simulink library "DareLib"  (R2018b)
settings: Solver=VariableStepAuto  StartTime=0.0  StopTime=10.0  RelTol=1e-3
libraries: simulink x4, $bdroot x3
(part 1 of 2)
settings Model: Creator=zhaogl  LastModifiedBy=Administrator

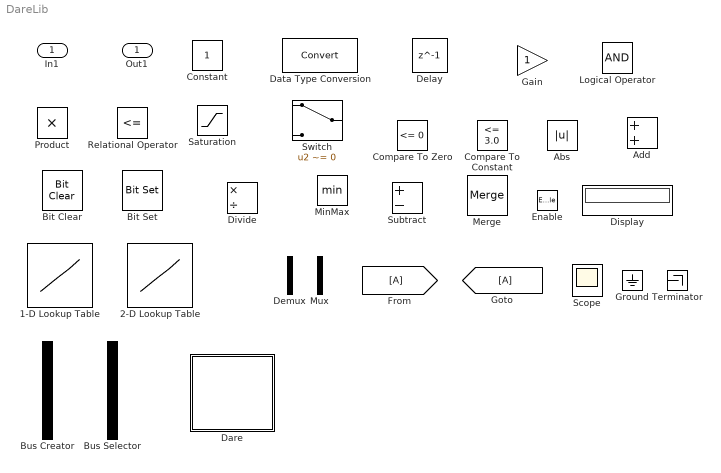
== system DareLib ==
  In1 : Inport
  Enable : EnablePort
      settings: AttributesFormatString=%<StatesWhenEnabling>
  1-D Lookup Table : Lookup_n-D  NumberOfTableDimensions=1  BreakpointsForDimension1=[-5:5]  Table=tanh([-5:5])  InternalRulePriority=Speed  RndMeth=Simplest  InputSameDT=on
  2-D Lookup Table : Lookup_n-D  BreakpointsForDimension1=[1:3]  BreakpointsForDimension2=[1:3]  InternalRulePriority=Speed  RndMeth=Simplest  InputSameDT=on
  Abs : Abs
  Add : Sum
  Bit Clear : simulink/Logic and Bit Operations/Bit Clear  iBit=0
      settings: SourceProductName=Simulink  SourceProductBaseCode=SL
  Bit Set : simulink/Logic and Bit Operations/Bit Set  iBit=0
      settings: SourceProductName=Simulink  SourceProductBaseCode=SL
  Bus Creator : BusCreator  Inputs=2
  Bus Selector : BusSelector  OutputSignals=signal1,signal2
  Compare To Constant : simulink/Logic and Bit Operations/Compare To Constant  relop=<=  const=3.0  OutDataTypeStr=boolean
  Compare To Zero : simulink/Logic and Bit Operations/Compare To Zero  relop=<=  OutDataTypeStr=boolean
  Constant : Constant
  Dare : Subsystem
      mask Display: image('Dare.jpg');
  Data Type Conversion : DataTypeConversion
  Delay : Delay  DelayLength=1  InitialCondition=0
  Demux : Demux  Outputs=2
  Display : Display
  Divide : Product  Inputs=*/
  Gain : Gain
  Ground : Ground
  Logical Operator : Logic  AllPortsSameDT=off  OutDataTypeStr=boolean
  Merge : Merge
  MinMax : MinMax
  Mux : Mux  Inputs=2
  Product : Product
  Relational Operator : RelationalOperator  Operator=<=  OutDataTypeStr=boolean  RndMeth=Simplest
  Saturation : Saturate
  Scope : Scope
  Subtract : Sum  Inputs=+-
  Switch : Switch  Criteria=u2 ~= 0
  Terminator : Terminator
  Out1 : Outport

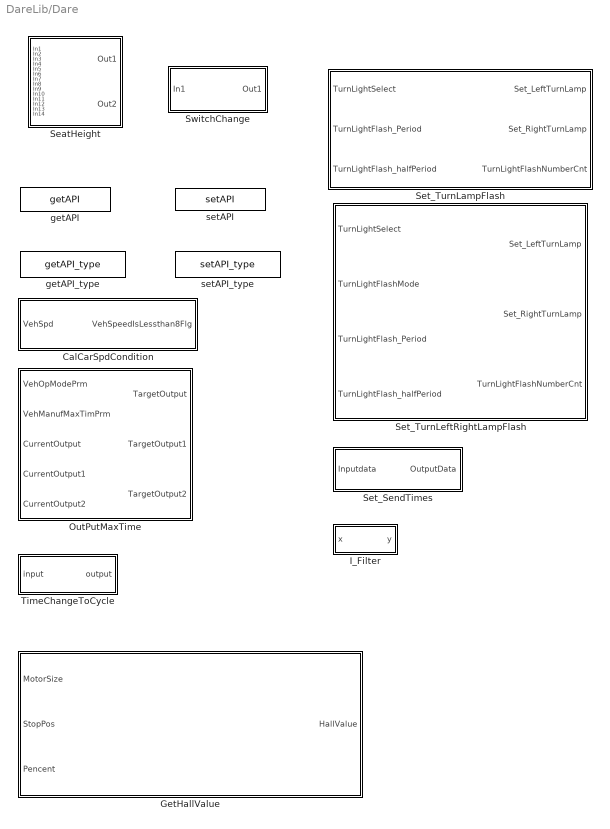
== system DareLib/Dare ==
  CalCarSpdCondition : Subsystem  mask(回差设定及判断){UpDeviationVal=9, DownDeviationVal=7, MaxOnTimer=500}
      mask prompts: UpDeviationVal "车速洄滞区间上限："; DownDeviationVal "车速洄滞区间下限："; MaxOnTimer "持续时间："
      mask help:
      | 功能描述
      | 车速判断回差，如雨刮速度模式的判断，当车速小于7km/h，持续时间5秒钟后，进入速度模式，大于9km/h持续时间5秒钟后退出速度模式，7~9km/h维持上次模式
      | 车速洄滞区间上限：如上述的9km/h
      | 车速洄滞区间下限：如上述的7km/h
      | 持续时间：如上述的5秒钟，需转成10ms单位，如5秒钟=5*1000/10=500
      mask Display:
      | port_label('input',1,'VehSpd','texmode','off');
      | 
      | 
      | port_label('output',1,'VehSpeedIsLessthan8Flg','texmode','off');
      | 
      | 
      | color('gray');
      | %disp('Dare');
      | text(0.14,0.8,'Dare','horizontalAlignment','right','verticalAlignment','bottom')
  GetHallValue : Subsystem
      settings: UndoDeleteFcn=Stateflow.SLINSF.SimulinkMan.restorePreDeleteFcn  PreDeleteFcn=Stateflow.SLINSF.SimulinkMan.removePreDeleteFcn
  I_Filter : Subsystem  mask(一阶滤波器){f=50}
      mask prompts: f "滤波系数："
      mask help: 用于信号滤波，滤波系数范围（0，100]，滤波系数越大，越接近输入值，滤波系数越小，曲线越平滑，根据实际需要选择不同滤波系数
      mask Display:
      | color('red');
      | disp(get_param(gcbh,'f'));
  OutPutMaxTime : Subsystem  Description=工厂模式限制输出时间  mask(OutPutMaxTime){UserMode=0, UnVaildValue=0}
      mask prompts: UserMode "用户模式值设定："; UnVaildValue "输出无效值设定："
      mask help: 在工厂模式和运输模式的最大工作时间设定，达到最大时间后输出无效值
      settings: AttributesFormatString=%<Description>
      mask Display:
      | port_label('input',1,'VehOpModePrm','texmode','off');
      | port_label('input',2,'VehManufMaxTimPrm','texmode','off');
      | port_label('input',3,'Input','texmode','off');
      | port_label('input',4,'Input1','texmode','off');
      | port_label('input',5,'Input2','texmode','off');
      | 
      | port_label('output',1,'Output','texmode','off');
      | port_label('output',2,'Output1','texmode','off');
      | port_label('output',3,'Output2','texmode','off');
      | 
      | 
      | color('gray')
      | text(0.11,0.94,'Dare','horizontalAlignment','right','verticalAlignment','bottom')
  SeatHeight : Subsystem
      mask help: 电动座椅控制封装函数
      mask Display: image('a.jpg');
  Set_SendTimes : Subsystem  mask(发送信号周期设定){Times=0}
      mask help:
      | InputSignal：输入发送信号
      | OnputSignal：输出发送信号
      | Times：设定发送信号不等于0时需要发送的帧数 (这实际是延迟周期数)，周期到后发送信号清零
      mask Display:
      | port_label('input',1,'InputSignal');
      | port_label('output',1,'OutputSignal');
      | 
      | color('gray');
      | %disp('Dare');
      | text(0.19,0.75,'Dare','horizontalAlignment','right','verticalAlignment','bottom')
  Set_TurnLampFlash : Subsystem  mask(控制转向灯闪烁及频率设定){TurnLight_Left=1, TurnLight_Right=2, TurnLight_LeftRight=3}
      mask prompts: TurnLight_Left "TurnLight_Left："; TurnLight_Right "TurnLight_Right："; TurnLight_LeftRight "TurnLight_LeftRight："
      mask help:
      | 第一个输入：TurnLightSelect：选择左右转向灯，enTurnLight_Left，enTurnLight_Right，enTurnLight_LeftRight
      | 第二个输入：TurnLightFlash_Period：闪烁周期设定
      | 第三个输入：TurnLightFlash_Period：闪烁周期内ON的时间设定
      | 参数设定，可根据实际修改：
      | TurnLight_Left：默认为1
      | TurnLight_Right：默认为2
      | TurnLight_LeftRight：默认为3
      mask Display:
      | port_label('input',1,'TurnLightSelect','texmode','off');
      | port_label('input',2,'TurnLightFlash_Period','texmode','off');
      | port_label('input',3,'TurnLightFlash_halfPeriod','texmode','off');
      | 
      | port_label('output',1,'Set_LeftTurnLamp','texmode','off');
      | port_label('output',2,'Set_RightTurnLamp','texmode','off');
      | port_label('output',3,'TurnLightFlashNumberCnt','texmode','off');
      | 
      | color('gray');
      | %disp('Dare');
      | text(0.09,0.93,'Dare','horizontalAlignment','right','verticalAlignment','bottom')
  Set_TurnLeftRightLampFlash : Subsystem  mask(控制转向灯闪烁频率设定及关闭){enTurnLight_Non=0, enTurnLight_Left=1, enTurnLight_Right=2, enTurnLight_LeftRight=3}
      mask prompts: enTurnLight_Non "TurnLight_Non"; enTurnLight_Left "TurnLight_Left"; enTurnLight_Right "TurnLight_Right"; enTurnLight_LeftRight "TurnLight_LeftRight"
      mask help:
      | 第一个输入：TurnLightSelect：选择左右转向灯，enTurnLight_Left，enTurnLight_Right，enTurnLight_LeftRight
      | 第二个输入：TurnLightFlashMode：ON为开启闪烁，OFF为关闭
      | 第三个输入：TurnLightFlash_Period：闪烁周期设定
      | 第四个输入：TurnLightFlash_Period：闪烁周期内ON的时间设定
      |
      | 参数设定：
      | enTurnLight_Non: 默认为0
      | enTurnLight_Left：默认为1
      | enTurnLight_Right：默认为2
      | enTurnLight_LeftRight：默认为3
      mask Display:
      | port_label('input',1,'TurnLightSelect','texmode','off');
      | port_label('input',2,'TurnLightFlashMode','texmode','off');
      | port_label('input',3,'TurnLightFlash_Period','texmode','off');
      | port_label('input',4,'TurnLightFlash_halfPeriod','texmode','off');
      | 
      | port_label('output',1,'Set_LeftTurnLamp','texmode','off');
      | port_label('output',2,'Set_RightTurnLamp','texmode','off');
      | port_label('output',3,'TurnLightFlashNumberCnt','texmode','off');
      | 
      | color('gray');
      | %disp('Dare');
      | text(0.12,0.96,'Dare','horizontalAlignment','right','verticalAlignment','bottom')
  SwitchChange : Subsystem  mask{d=1, a=0, b=1, c=2}
      mask prompts: d "设置开关有效："; a "状态  保持："; b "无效变有效："; c "有效变无效："
      mask help:
      | 检测自复位开关有效变化
      | 设置开关有效：如1有效则填1，2有效则填2
      mask Display:
      | disp('Reset Switch')
      | 
      | color('gray')
      | text(0.25,0.8,'Dare','horizontalAlignment','right','verticalAlignment','bottom')
  TimeChangeToCycle : Subsystem  Description=时间转成执行周期  mask{Sec=1, Msec=1000, Cycle=10}
      mask prompts: Sec "秒参数设定："; Msec "毫秒参数设定："; Cycle "执行周期设定："
      mask help:
      | y=x*sec*msec/cycle，通过时间计算执行周期
      | 秒参数设定：如果目标是分，填60s，如果目标是秒，填1，就是把分换算成秒
      | 毫秒参数设定：把秒换算成分，1s=1000ms
      | 执行周期设定：当前模型执行的周期
      settings: AttributesFormatString=%<Description>
      mask Display:
      | port_label('input',1,'input','texmode','off');
      | port_label('output',1,'output','texmode','off');
      | 
      | color('gray')
      | %disp('Dare');
      | text(0.25,0.75,'Dare','horizontalAlignment','right','verticalAlignment','bottom')
  getAPI : S-Function  FunctionName=getAPI  Parameters=g_funcname,g_param,g_type  SFunctionDeploymentMode=off  EnableBusSupport=off  mask(Dare Custom){g_funcname=getAPI, g_param=, g_type=uint8}
      mask prompts: g_funcname "API function name:"; g_param "API        param:"; g_type "API OutPut Type:"
      mask help:
      | This block generates get interface function API.
      | function name : Enter the interface function name.
      | param : Input interface function parameters
      | type :  choose The interface function returns the type
      settings: AttributesFormatString=%<g_funcname>
      mask TypeOptions g_type: boolean | uint8 | int8 | uint16 | int16 | uint32 | int32
      mask Display:
      | %color('green')
      | 
      | if isempty(g_param)
      |     %disp(get_param(gcbh,'g_funcname'));
      | else
      |     disp(get_param(gcbh,'g_param'));
      | end
      | %text(0.01,0.8,get_param(gcbh,'g_funcname'))
      | %text(0.6,0.2,get_param(gcbh,'g_param'))
      | 
      | color('gray')
      | text(0.25,0.63,'Dare','horizontalAlignment','right','verticalAlignment','bottom')
  getAPI_type : S-Function  FunctionName=getAPI_type  Parameters=g_funcname,g_param,g_type,g_enum,g_size  SFunctionDeploymentMode=off  EnableBusSupport=off  mask(Dare Custom){g_funcname=getAPI_type, g_param=, g_type=uint8, g_enum=, g_size=-1}
      mask prompts: g_funcname "API  Function Name:"; g_param "API  Param:"; g_type "API Output Type:"; g_enum "API Output Type Enum:"; g_size "API  Dimensions:"
      mask help:
      | This block generates get interface function API.
      | function name : Enter the interface function name.
      | param : Input interface function parameters
      | type :  choose The interface function returns the type
      | enum: choose enum type
      settings: AttributesFormatString=%<g_funcname>
      mask TypeOptions g_type: boolean | int8 | uint8 | int16 | uint16 | int32 | uint32 | double
      mask TypeOptions g_enum: ExitGearCause | enAdjustEnable | enBackGear | enDrAdjustEnable | enEngineType | enFinalPowerMode | enFrontGear | enHeatCmdFault | enHeatIoCmdLvl | enHeatIoSts | enHeatLvlSts | enHeatNtcFault | enHeatStopReason | enHeatType | enIgnSts | enLearnCmd | enLearnExitCause | enLearnSts | enLengthGear | enMasReason | enMassageLevel_DSM | enMassageLevel_IVI | enMassageMode_DSM | enMassageMode_IVI | enMemBtn | enMemCallFb | enMemSet | enMemSetFb | enMemStopCause | enMotorLearn | enNapMode | enPowerModeSts | enProjectType | enResCallRet | enResetSts | enSWMoveCmd | enSeatAutoRunSts | enSeatHightMotorRunsts | enSeatMemBtnCmd | enSeatMemBtnSts | enSeatMemStsAndMsg | enSeatMemStsFb | enSeatMotorRunTye | enSeatMotorRunType | enSeatMoveCmd | enSoftStopFault | enSteerHeatType | enSystemVolt | enTcmGearLvlSts | enVehTypePrm | enVehicleRunType | enVentCmdFault | enVentIoCmdLvl | enVentLvlSts | enVentStopReason | enVentType | enVoltageMode | enWelStopCause | enWelcomeRunSts | enWelcomeSts
      mask Display:
      | %color('green')
      | 
      | if isempty(g_param)
      |     %disp(get_param(gcbh,'g_funcname'));
      | else
      |     disp(get_param(gcbh,'g_param'));
      | end
      | %text(0.01,0.8,get_param(gcbh,'g_funcname'))
      | %text(0.6,0.2,get_param(gcbh,'g_param'))
      | 
      | color('gray')
      | text(0.25,0.63,'Dare','horizontalAlignment','right','verticalAlignment','bottom')
      | 
      | if isempty(get_param(gcbh,'g_enum'))
      |     set_param(gcbh','MaskVisibilityString', 'on,on,on,on,on')
      | else
      |     set_param(gcbh','MaskVisibilityString', 'on,on,off,on,on')
      | end
  setAPI : S-Function  FunctionName=setAPI  Parameters=g_funcname,g_param,g_type  SFunctionDeploymentMode=off  EnableBusSupport=off  mask(Dare Custom){g_funcname=setAPI, g_param=, g_type=uint8}
      mask prompts: g_funcname "API function name:"; g_param "API         param:"; g_type "API OutPut Type:"
      mask help:
      | This block generates set interface function API.
      | function name : Enter the interface function name.
      | API function param : Input interface function parameters
      | API param：choose channel number
      | type :  choose The interface function returns the type
      settings: AttributesFormatString=%<g_funcname>
      mask TypeOptions g_type: boolean | uint8 | int8 | uint16 | int16 | uint32 | int32 | double
      mask Display:
      | %color('magenta')
      | %disp(get_param(gcbh,'g_param'))
      | if isempty(g_param)
      |     %disp(get_param(gcbh,'g_funcname'));
      | else
      |     disp(get_param(gcbh,'g_param'));
      | end
      | 
      | color('gray')
      | text(0.25,0.61,'Dare','horizontalAlignment','right','verticalAlignment','bottom')
  setAPI_type : S-Function  FunctionName=setAPI_type  Parameters=g_funcname,g_param,g_type,g_enum,g_size  SFunctionDeploymentMode=off  EnableBusSupport=off  mask(Dare Custom){g_funcname=setAPI_type, g_param=, g_type=uint8, g_enum=, g_size=-1}
      mask prompts: g_funcname "API  Function Name:"; g_param "API  Param:"; g_type "API Output Type:"; g_enum "API Output Type Enum:"; g_size "API  Dimensions:"
      mask help:
      | This block generates get interface function API.
      | function name : Enter the interface function name.
      | param : Input interface function parameters
      | type :  choose The interface function returns the type
      | enum: choose enum type
      settings: AttributesFormatString=%<g_funcname>
      mask TypeOptions g_type: boolean | int8 | uint8 | int16 | uint16 | int32 | uint32 | double
      mask TypeOptions g_enum: ExitGearCause | enAdjustEnable | enBackGear | enDrAdjustEnable | enEngineType | enFinalPowerMode | enFrontGear | enHeatCmdFault | enHeatIoCmdLvl | enHeatIoSts | enHeatLvlSts | enHeatNtcFault | enHeatStopReason | enHeatType | enIgnSts | enLearnCmd | enLearnExitCause | enLearnSts | enLengthGear | enMasReason | enMassageLevel_DSM | enMassageLevel_IVI | enMassageMode_DSM | enMassageMode_IVI | enMemBtn | enMemCallFb | enMemSet | enMemSetFb | enMemStopCause | enMotorLearn | enNapMode | enPowerModeSts | enProjectType | enResCallRet | enResetSts | enSWMoveCmd | enSeatAutoRunSts | enSeatHightMotorRunsts | enSeatMemBtnCmd | enSeatMemBtnSts | enSeatMemStsAndMsg | enSeatMemStsFb | enSeatMotorRunTye | enSeatMotorRunType | enSeatMoveCmd | enSoftStopFault | enSteerHeatType | enSystemVolt | enTcmGearLvlSts | enVehTypePrm | enVehicleRunType | enVentCmdFault | enVentIoCmdLvl | enVentLvlSts | enVentStopReason | enVentType | enVoltageMode | enWelStopCause | enWelcomeRunSts | enWelcomeSts
      mask Display:
      | %color('green')
      | 
      | if isempty(get_param(gcbh,'g_param'))
      |     %disp(get_param(gcbh,'g_funcname'));
      | else
      |     disp(get_param(gcbh,'g_param'));
      | end
      | %text(0.01,0.8,get_param(gcbh,'g_funcname'))
      | %text(0.6,0.2,get_param(gcbh,'g_param'))
      | 
      | color('gray')
      | text(0.25,0.63,'Dare','horizontalAlignment','right','verticalAlignment','bottom')
      | 
      | if isempty(get_param(gcbh,'g_enum'))
      |     set_param(gcbh','MaskVisibilityString', 'on,on,on,on,on')
      | else
      |     set_param(gcbh','MaskVisibilityString', 'on,on,off,on,on')
      | end

== system DareLib/Dare/CalCarSpdCondition ==
  " VehSpd" : Inport
  Chart : Stateflow chart  TreatAsAtomicUnit=on
  Constant : Constant  Value=UpDeviationVal  OutDataTypeStr=uint8
  Constant2 : Constant  Value=DownDeviationVal  OutDataTypeStr=uint8
  Constant3 : Constant  Value=MaxOnTimer  OutDataTypeStr=uint16
  VehSpeedIsLessthan8Flg : Outport
  wires:
  " VehSpd"/1 -> Chart/1(VehSpd)
  Constant3/1 -> Chart/4(CAL_MaxOnTimer)
  Chart/1(VehSpdUpDnFlg) -> VehSpeedIsLessthan8Flg/1
  Constant/1 -> Chart/3(UpVal)
  Constant2/1 -> Chart/2(DnVal)

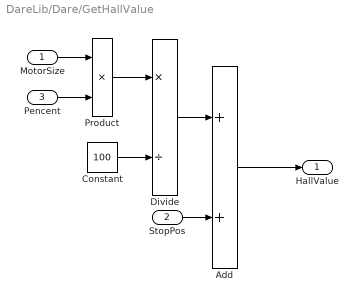
== system DareLib/Dare/GetHallValue ==
  MotorSize : Inport  OutDataTypeStr=uint16
  StopPos : Inport  Port=2  OutDataTypeStr=uint16
  Pencent : Inport  Port=3  OutDataTypeStr=uint8
  Add : Sum  AccumDataTypeStr=uint16
  Constant : Constant  Value=100  OutDataTypeStr=uint16
  Divide : Product  Inputs=*/  OutDataTypeStr=uint16
  Product : Product  OutDataTypeStr=uint32
  HallValue : Outport  OutDataTypeStr=uint16
  wires:
  Divide/1 -> Add/1
  Constant/1 -> Divide/2
  Product/1 -> Divide/1
  Pencent/1 -> Product/2
  StopPos/1 -> Add/2
  MotorSize/1 -> Product/1
  Add/1 -> HallValue/1

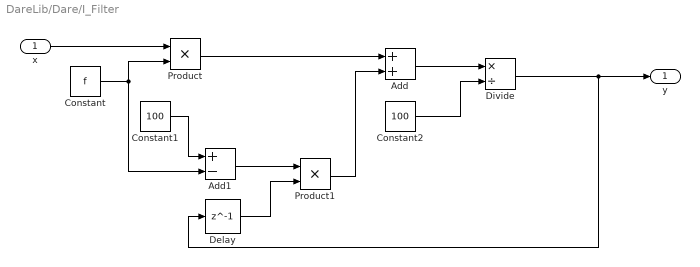
== system DareLib/Dare/I_Filter ==
  x : Inport
  Add : Sum
  Add1 : Sum  Inputs=+-
  Constant : Constant  Value=f  OutDataTypeStr=uint8
  Constant1 : Constant  Value=100  OutDataTypeStr=uint8
  Constant2 : Constant  Value=100  OutDataTypeStr=uint8
  Delay : Delay  DelayLength=1  InitialCondition=0
  Divide : Product  Inputs=*/
  Product : Product
  Product1 : Product  OutDataTypeStr=uint32
  y : Outport
  wires:
  Constant2/1 -> Divide/2
  Add/1 -> Divide/1
  Add1/1 -> Product1/1
  Product/1 -> Add/1
  Delay/1 -> Product1/2
  Product1/1 -> Add/2
  Divide/1 -> Delay/1, y/1
  x/1 -> Product/1
  Constant1/1 -> Add1/1
  Constant/1 -> Product/2, Add1/2

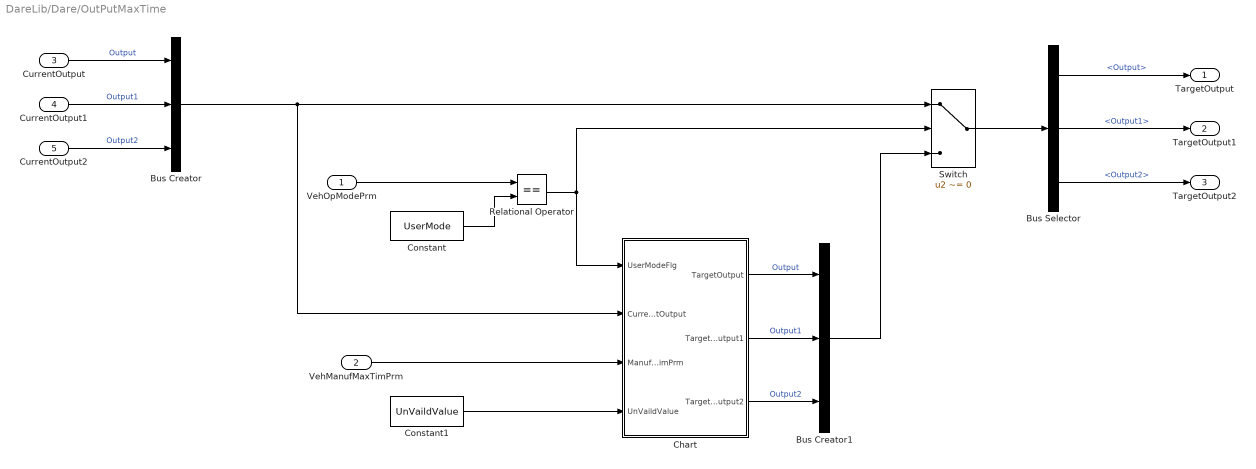
== system DareLib/Dare/OutPutMaxTime ==
  VehOpModePrm : Inport
  VehManufMaxTimPrm : Inport  Port=2
  CurrentOutput : Inport  Port=3
  CurrentOutput1 : Inport  Port=4
  CurrentOutput2 : Inport  Port=5
  Bus Creator : BusCreator  Inputs=3
  Bus Creator1 : BusCreator  Inputs=3
  Bus Selector : BusSelector  OutputSignals=Output,Output1,Output2
  Chart : Stateflow chart  TreatAsAtomicUnit=on
  Constant : Constant  Value=UserMode  OutDataTypeStr=uint8
  Constant1 : Constant  Value=UnVaildValue  OutDataTypeStr=uint8
  Relational Operator : RelationalOperator  Operator===  OutDataTypeStr=boolean  RndMeth=Simplest
  Switch : Switch  Criteria=u2 ~= 0
  TargetOutput : Outport
  TargetOutput1 : Outport  Port=2
  TargetOutput2 : Outport  Port=3
  wires:
  Constant1/1 -> Chart/4(UnVaildValue)
  Relational Operator/1 -> Chart/1(UserModeFlg), Switch/2
  VehManufMaxTimPrm/1 -> Chart/3(ManufMaxTimPrm)
  Constant/1 -> Relational Operator/2
  Bus Creator/1 -> Chart/2(CurrentOutput), Switch/1
  VehOpModePrm/1 -> Relational Operator/1
  CurrentOutput/1 -> Bus Creator/1  "Output"
  CurrentOutput1/1 -> Bus Creator/2  "Output1"
  CurrentOutput2/1 -> Bus Creator/3  "Output2"
  Chart/3(TargetOutput2) -> Bus Creator1/3  "Output2"
  Chart/1(TargetOutput) -> Bus Creator1/1  "Output"
  Bus Creator1/1 -> Switch/3
  Chart/2(TargetOutput1) -> Bus Creator1/2  "Output1"
  Bus Selector/2 -> TargetOutput1/1  "<Output1>"
  Bus Selector/1 -> TargetOutput/1  "<Output>"
  Switch/1 -> Bus Selector/1
  Bus Selector/3 -> TargetOutput2/1  "<Output2>"

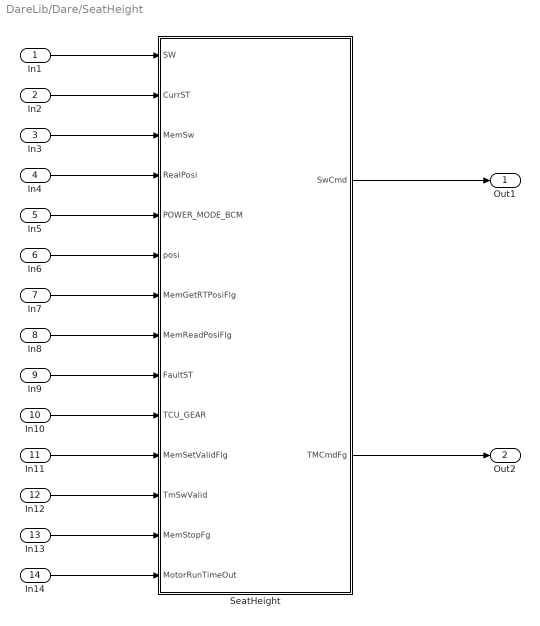
== system DareLib/Dare/SeatHeight ==
  In1 : Inport
  In2 : Inport  Port=2
  In3 : Inport  Port=3
  In4 : Inport  Port=4
  In5 : Inport  Port=5
  In6 : Inport  Port=6
  In7 : Inport  Port=7
  In8 : Inport  Port=8
  In9 : Inport  Port=9
  In10 : Inport  Port=10
  In11 : Inport  Port=11
  In12 : Inport  Port=12
  In13 : Inport  Port=13
  In14 : Inport  Port=14
  SeatHeight : Stateflow chart  TreatAsAtomicUnit=on
  Out1 : Outport
  Out2 : Outport  Port=2
  wires:
  In4/1 -> SeatHeight/4(RealPosi)
  In5/1 -> SeatHeight/5(POWER_MODE_BCM)
  In7/1 -> SeatHeight/7(MemGetRTPosiFlg)
  In8/1 -> SeatHeight/8(MemReadPosiFlg)
  SeatHeight/1(SwCmd) -> Out1/1
  In3/1 -> SeatHeight/3(MemSw)
  In6/1 -> SeatHeight/6(posi)
  In1/1 -> SeatHeight/1(SW)
  In9/1 -> SeatHeight/9(FaultST)
  In2/1 -> SeatHeight/2(CurrST)
  In12/1 -> SeatHeight/12(TmSwValid)
  In10/1 -> SeatHeight/10(TCU_GEAR)
  In11/1 -> SeatHeight/11(MemSetValidFlg)
  In14/1 -> SeatHeight/14(MotorRunTimeOut)
  In13/1 -> SeatHeight/13(MemStopFg)
  SeatHeight/2(TMCmdFg) -> Out2/1

== system DareLib/Dare/Set_SendTimes ==
  Inputdata : Inport
  Chart : Stateflow chart  TreatAsAtomicUnit=on
  Times : Constant  Value=Times  OutDataTypeStr=uint8
  OutputData : Outport
  wires:
  Inputdata/1 -> Chart/1(Inputdata)
  Times/1 -> Chart/2(Times)
  Chart/1(OutputData) -> OutputData/1

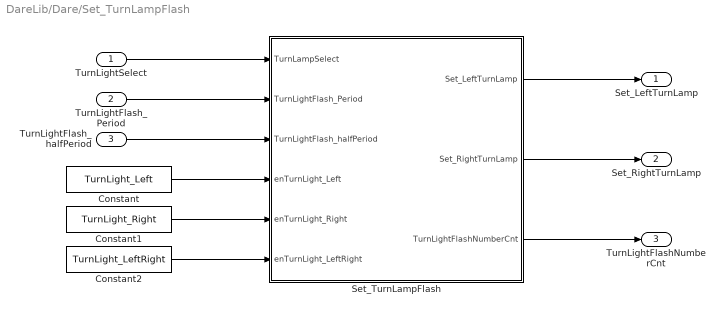
== system DareLib/Dare/Set_TurnLampFlash ==
  TurnLightSelect : Inport
  TurnLightFlash_Period : Inport  Port=2
  TurnLightFlash_halfPeriod : Inport  Port=3
  Constant : Constant  Value=TurnLight_Left  OutDataTypeStr=uint8
  Constant1 : Constant  Value=TurnLight_Right  OutDataTypeStr=uint8
  Constant2 : Constant  Value=TurnLight_LeftRight  OutDataTypeStr=uint8
  Set_TurnLampFlash : Stateflow chart  TreatAsAtomicUnit=on
  Set_LeftTurnLamp : Outport
  Set_RightTurnLamp : Outport  Port=2
  TurnLightFlashNumberCnt : Outport  Port=3
  wires:
  Constant/1 -> Set_TurnLampFlash/4(enTurnLight_Left)
  Constant1/1 -> Set_TurnLampFlash/5(enTurnLight_Right)
  Constant2/1 -> Set_TurnLampFlash/6(enTurnLight_LeftRight)
  TurnLightFlash_Period/1 -> Set_TurnLampFlash/2(TurnLightFlash_Period)
  Set_TurnLampFlash/2(Set_RightTurnLamp) -> Set_RightTurnLamp/1
  Set_TurnLampFlash/1(Set_LeftTurnLamp) -> Set_LeftTurnLamp/1
  TurnLightSelect/1 -> Set_TurnLampFlash/1(TurnLampSelect)
  TurnLightFlash_halfPeriod/1 -> Set_TurnLampFlash/3(TurnLightFlash_halfPeriod)
  Set_TurnLampFlash/3(TurnLightFlashNumberCnt) -> TurnLightFlashNumberCnt/1

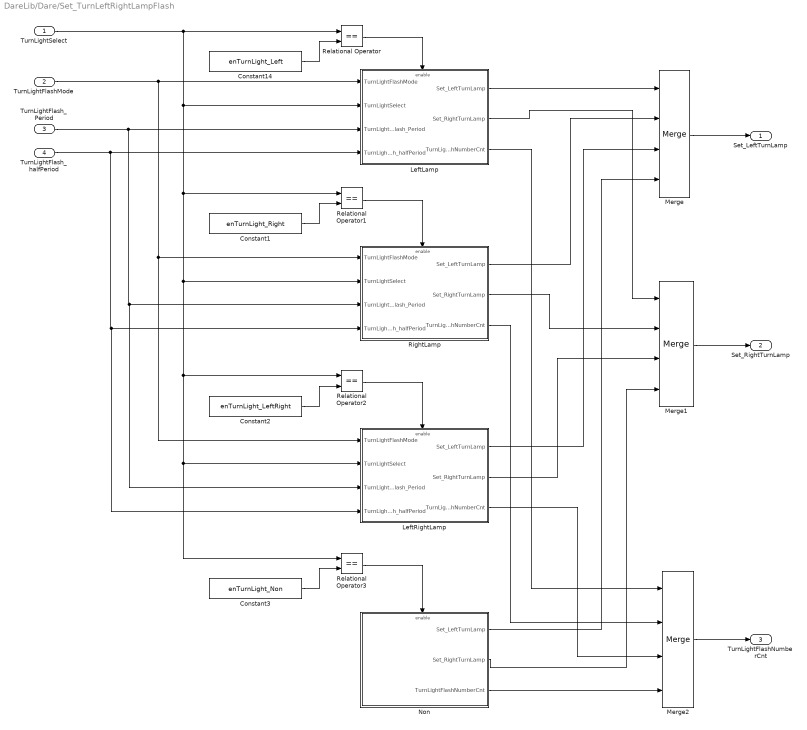
== system DareLib/Dare/Set_TurnLeftRightLampFlash ==
  TurnLightSelect : Inport
  TurnLightFlashMode : Inport  Port=2
  TurnLightFlash_Period : Inport  Port=3
  TurnLightFlash_halfPeriod : Inport  Port=4
  Constant1 : Constant  Value=enTurnLight_Right  OutDataTypeStr=uint8
  Constant14 : Constant  Value=enTurnLight_Left  OutDataTypeStr=uint8
  Constant2 : Constant  Value=enTurnLight_LeftRight  OutDataTypeStr=uint8
  Constant3 : Constant  Value=enTurnLight_Non  OutDataTypeStr=uint8
  LeftLamp : Subsystem  TreatAsAtomicUnit=on
  LeftRightLamp : Subsystem  TreatAsAtomicUnit=on
  Merge : Merge  Inputs=4
  Merge1 : Merge  Inputs=4
  Merge2 : Merge  Inputs=4
  Non : Subsystem  TreatAsAtomicUnit=on
  Relational Operator{,1..3} (4 alike) : RelationalOperator  Operator===  OutDataTypeStr=boolean  RndMeth=Simplest
  RightLamp : Subsystem  TreatAsAtomicUnit=on
  Set_LeftTurnLamp : Outport
  Set_RightTurnLamp : Outport  Port=2
  TurnLightFlashNumberCnt : Outport  Port=3
  wires:
  LeftLamp/2(Set_RightTurnLamp) -> Merge1/1
  Relational Operator1/1 -> RightLamp/Enable
  Constant1/1 -> Relational Operator1/2
  Relational Operator/1 -> LeftLamp/Enable
  RightLamp/3(TurnLightFlashNumberCnt) -> Merge2/2
  Constant14/1 -> Relational Operator/2
  Constant2/1 -> Relational Operator2/2
  Relational Operator2/1 -> LeftRightLamp/Enable
  LeftLamp/3(TurnLightFlashNumberCnt) -> Merge2/1
  RightLamp/2(Set_RightTurnLamp) -> Merge1/2
  LeftRightLamp/1(Set_LeftTurnLamp) -> Merge/3
  Merge/1 -> Set_LeftTurnLamp/1
  Merge1/1 -> Set_RightTurnLamp/1
  LeftLamp/1(Set_LeftTurnLamp) -> Merge/1
  LeftRightLamp/2(Set_RightTurnLamp) -> Merge1/3
  LeftRightLamp/3(TurnLightFlashNumberCnt) -> Merge2/3
  Merge2/1 -> TurnLightFlashNumberCnt/1
  RightLamp/1(Set_LeftTurnLamp) -> Merge/2
  TurnLightFlash_Period/1 -> LeftRightLamp/3(TurnLightFlash_Period), RightLamp/3(TurnLightFlash_Period), LeftLamp/3(TurnLightFlash_Period)
  Relational Operator3/1 -> Non/Enable
  Constant3/1 -> Relational Operator3/2
  TurnLightFlash_halfPeriod/1 -> LeftRightLamp/4(TurnLightFlash_halfPeriod), RightLamp/4(TurnLightFlash_halfPeriod), LeftLamp/4(TurnLightFlash_halfPeriod)
  TurnLightSelect/1 -> LeftLamp/2(TurnLightSelect), RightLamp/2(TurnLightSelect), Relational Operator3/1, LeftRightLamp/2(TurnLightSelect), Relational Operator2/1, Relational Operator1/1, Relational Operator/1
  TurnLightFlashMode/1 -> LeftRightLamp/1(TurnLightFlashMode), RightLamp/1(TurnLightFlashMode), LeftLamp/1(TurnLightFlashMode)
  Non/3(TurnLightFlashNumberCnt) -> Merge2/4
  Non/1(Set_LeftTurnLamp) -> Merge/4
  Non/2(Set_RightTurnLamp) -> Merge1/4

== system DareLib/Dare/SwitchChange ==
  In1 : Inport
  ButtonChange : Stateflow chart  TreatAsAtomicUnit=on
  Constant1 : Constant  Value=d  OutDataTypeStr=uint8
  Constant2 : Constant  Value=a  OutDataTypeStr=uint8
  Constant3 : Constant  Value=b  OutDataTypeStr=uint8
  Constant4 : Constant  Value=c  OutDataTypeStr=uint8
  Out1 : Outport
  wires:
  Constant2/1 -> ButtonChange/2(enSw_NoChanged)
  In1/1 -> ButtonChange/1(CurSw)
  Constant4/1 -> ButtonChange/4(enSw_ValidToUnvalid)
  Constant3/1 -> ButtonChange/3(enSw_UnvalidToValid)
  ButtonChange/1(SwSts) -> Out1/1
  Constant1/1 -> ButtonChange/5(Vaild_Vaule)

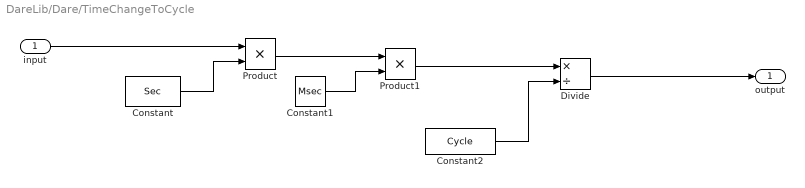
== system DareLib/Dare/TimeChangeToCycle ==
  input : Inport
  Constant : Constant  Value=Sec  OutDataTypeStr=uint16
  Constant1 : Constant  Value=Msec  OutDataTypeStr=uint16
  Constant2 : Constant  Value=Cycle  OutDataTypeStr=uint8
  Divide : Product  Inputs=*/  OutDataTypeStr=uint32
  Product : Product
  Product1 : Product  OutDataTypeStr=uint32
  output : Outport
  wires:
  Constant2/1 -> Divide/2
  Product/1 -> Product1/1
  Constant1/1 -> Product1/2
  Product1/1 -> Divide/1
  Constant/1 -> Product/2
  input/1 -> Product/1
  Divide/1 -> output/1

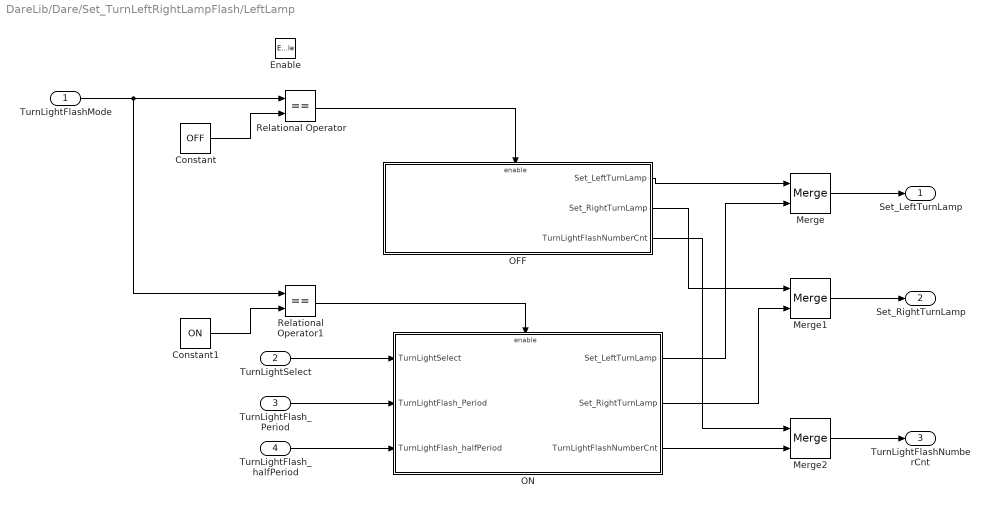
== system DareLib/Dare/Set_TurnLeftRightLampFlash/LeftLamp ==
  TurnLightFlashMode : Inport
  TurnLightSelect : Inport  Port=2
  TurnLightFlash_Period : Inport  Port=3
  TurnLightFlash_halfPeriod : Inport  Port=4
  Enable : EnablePort
  Constant : Constant  Value=OFF  OutDataTypeStr=uint8
  Constant1 : Constant  Value=ON  OutDataTypeStr=uint8
  Merge : Merge
  Merge1 : Merge
  Merge2 : Merge
  OFF : Subsystem  TreatAsAtomicUnit=on
  ON : Subsystem  TreatAsAtomicUnit=on
  Relational Operator : RelationalOperator  Operator===  OutDataTypeStr=boolean  RndMeth=Simplest
  Relational Operator1 : RelationalOperator  Operator===  OutDataTypeStr=boolean  RndMeth=Simplest
  Set_LeftTurnLamp : Outport
  Set_RightTurnLamp : Outport  Port=2
  TurnLightFlashNumberCnt : Outport  Port=3
  wires:
  Relational Operator/1 -> OFF/Enable
  Constant/1 -> Relational Operator/2
  Constant1/1 -> Relational Operator1/2
  Relational Operator1/1 -> ON/Enable
  TurnLightFlashMode/1 -> Relational Operator1/1, Relational Operator/1
  OFF/1(Set_LeftTurnLamp) -> Merge/1
  ON/1(Set_LeftTurnLamp) -> Merge/2
  OFF/2(Set_RightTurnLamp) -> Merge1/1
  ON/2(Set_RightTurnLamp) -> Merge1/2
  Merge/1 -> Set_LeftTurnLamp/1
  Merge1/1 -> Set_RightTurnLamp/1
  TurnLightSelect/1 -> ON/1(TurnLightSelect)
  TurnLightFlash_Period/1 -> ON/2(TurnLightFlash_Period)
  TurnLightFlash_halfPeriod/1 -> ON/3(TurnLightFlash_halfPeriod)
  Merge2/1 -> TurnLightFlashNumberCnt/1
  OFF/3(TurnLightFlashNumberCnt) -> Merge2/1
  ON/3(TurnLightFlashNumberCnt) -> Merge2/2

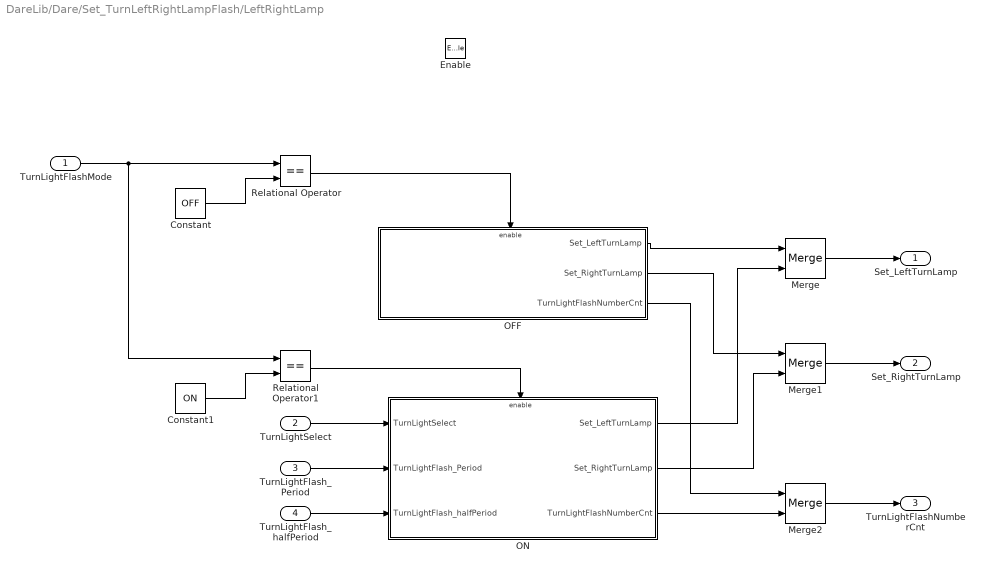
== system DareLib/Dare/Set_TurnLeftRightLampFlash/LeftRightLamp ==
  TurnLightFlashMode : Inport
  TurnLightSelect : Inport  Port=2
  TurnLightFlash_Period : Inport  Port=3
  TurnLightFlash_halfPeriod : Inport  Port=4
  Enable : EnablePort
  Constant : Constant  Value=OFF
  Constant1 : Constant  Value=ON
  Merge : Merge
  Merge1 : Merge
  Merge2 : Merge
  OFF : Subsystem  TreatAsAtomicUnit=on
  ON : Subsystem  TreatAsAtomicUnit=on
  Relational Operator : RelationalOperator  Operator===  OutDataTypeStr=boolean  RndMeth=Simplest
  Relational Operator1 : RelationalOperator  Operator===  OutDataTypeStr=boolean  RndMeth=Simplest
  Set_LeftTurnLamp : Outport
  Set_RightTurnLamp : Outport  Port=2
  TurnLightFlashNumberCnt : Outport  Port=3
  wires:
  Constant/1 -> Relational Operator/2
  Relational Operator1/1 -> ON/Enable
  Relational Operator/1 -> OFF/Enable
  Constant1/1 -> Relational Operator1/2
  TurnLightFlashMode/1 -> Relational Operator1/1, Relational Operator/1
  Merge/1 -> Set_LeftTurnLamp/1
  ON/2(Set_RightTurnLamp) -> Merge1/2
  OFF/1(Set_LeftTurnLamp) -> Merge/1
  OFF/2(Set_RightTurnLamp) -> Merge1/1
  Merge1/1 -> Set_RightTurnLamp/1
  ON/1(Set_LeftTurnLamp) -> Merge/2
  TurnLightSelect/1 -> ON/1(TurnLightSelect)
  TurnLightFlash_Period/1 -> ON/2(TurnLightFlash_Period)
  TurnLightFlash_halfPeriod/1 -> ON/3(TurnLightFlash_halfPeriod)
  ON/3(TurnLightFlashNumberCnt) -> Merge2/2
  OFF/3(TurnLightFlashNumberCnt) -> Merge2/1
  Merge2/1 -> TurnLightFlashNumberCnt/1

== system DareLib/Dare/Set_TurnLeftRightLampFlash/Non ==
  Enable : EnablePort
  Constant : Constant  Value=0  OutDataTypeStr=uint8
  Constant1 : Constant  Value=0  OutDataTypeStr=uint8
  Constant2 : Constant  Value=0  OutDataTypeStr=uint16
  Set_LeftTurnLamp : Outport
  Set_RightTurnLamp : Outport  Port=2
  TurnLightFlashNumberCnt : Outport  Port=3
  wires:
  Constant1/1 -> Set_RightTurnLamp/1
  Constant/1 -> Set_LeftTurnLamp/1
  Constant2/1 -> TurnLightFlashNumberCnt/1

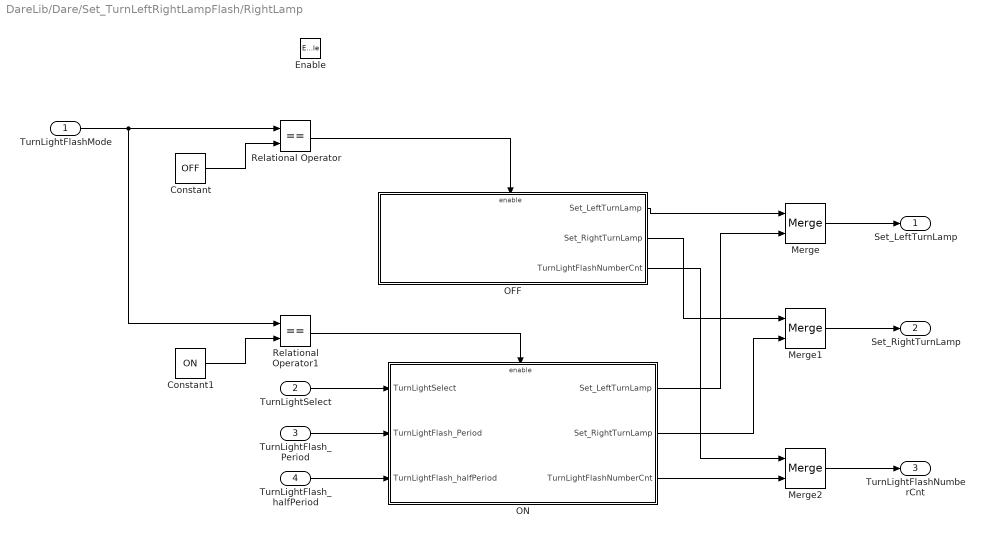
== system DareLib/Dare/Set_TurnLeftRightLampFlash/RightLamp ==
  TurnLightFlashMode : Inport
  TurnLightSelect : Inport  Port=2
  TurnLightFlash_Period : Inport  Port=3
  TurnLightFlash_halfPeriod : Inport  Port=4
  Enable : EnablePort
  Constant : Constant  Value=OFF
  Constant1 : Constant  Value=ON
  Merge : Merge
  Merge1 : Merge
  Merge2 : Merge
  OFF : Subsystem  TreatAsAtomicUnit=on
  ON : Subsystem  TreatAsAtomicUnit=on
  Relational Operator : RelationalOperator  Operator===  OutDataTypeStr=boolean  RndMeth=Simplest
  Relational Operator1 : RelationalOperator  Operator===  OutDataTypeStr=boolean  RndMeth=Simplest
  Set_LeftTurnLamp : Outport
  Set_RightTurnLamp : Outport  Port=2
  TurnLightFlashNumberCnt : Outport  Port=3
  wires:
  TurnLightFlashMode/1 -> Relational Operator1/1, Relational Operator/1
  Relational Operator1/1 -> ON/Enable
  Constant1/1 -> Relational Operator1/2
  Constant/1 -> Relational Operator/2
  Relational Operator/1 -> OFF/Enable
  Merge/1 -> Set_LeftTurnLamp/1
  ON/2(Set_RightTurnLamp) -> Merge1/2
  OFF/1(Set_LeftTurnLamp) -> Merge/1
  OFF/2(Set_RightTurnLamp) -> Merge1/1
  Merge1/1 -> Set_RightTurnLamp/1
  ON/1(Set_LeftTurnLamp) -> Merge/2
  TurnLightSelect/1 -> ON/1(TurnLightSelect)
  TurnLightFlash_Period/1 -> ON/2(TurnLightFlash_Period)
  TurnLightFlash_halfPeriod/1 -> ON/3(TurnLightFlash_halfPeriod)
  Merge2/1 -> TurnLightFlashNumberCnt/1
  OFF/3(TurnLightFlashNumberCnt) -> Merge2/1
  ON/3(TurnLightFlashNumberCnt) -> Merge2/2

== system DareLib/Dare/Set_TurnLeftRightLampFlash/LeftLamp/OFF ==
  Enable : EnablePort
  Constant : Constant  Value=0  OutDataTypeStr=uint8
  Constant1 : Constant  Value=0  OutDataTypeStr=uint8
  Constant2 : Constant  Value=0  OutDataTypeStr=uint16
  Set_LeftTurnLamp : Outport
  Set_RightTurnLamp : Outport  Port=2
  TurnLightFlashNumberCnt : Outport  Port=3
  wires:
  Constant/1 -> Set_LeftTurnLamp/1
  Constant1/1 -> Set_RightTurnLamp/1
  Constant2/1 -> TurnLightFlashNumberCnt/1

== system DareLib/Dare/Set_TurnLeftRightLampFlash/LeftLamp/ON ==
  TurnLightSelect : Inport
  TurnLightFlash_Period : Inport  Port=2
  TurnLightFlash_halfPeriod : Inport  Port=3
  Enable : EnablePort  StatesWhenEnabling=reset
      settings: AttributesFormatString=%<StatesWhenEnabling>
  Set_TurnLampFlash : $bdroot/Dare/Set_TurnLampFlash  TurnLight_Left=1  TurnLight_Right=2  TurnLight_LeftRight=3
  Set_LeftTurnLamp : Outport
  Set_RightTurnLamp : Outport  Port=2
  TurnLightFlashNumberCnt : Outport  Port=3
  wires:
  TurnLightSelect/1 -> Set_TurnLampFlash/1
  TurnLightFlash_Period/1 -> Set_TurnLampFlash/2
  TurnLightFlash_halfPeriod/1 -> Set_TurnLampFlash/3
  Set_TurnLampFlash/1 -> Set_LeftTurnLamp/1
  Set_TurnLampFlash/2 -> Set_RightTurnLamp/1
  Set_TurnLampFlash/3 -> TurnLightFlashNumberCnt/1

== system DareLib/Dare/Set_TurnLeftRightLampFlash/LeftRightLamp/OFF ==
  Enable : EnablePort
  Constant : Constant  Value=0  OutDataTypeStr=uint8
  Constant1 : Constant  Value=0  OutDataTypeStr=uint8
  Constant2 : Constant  Value=0  OutDataTypeStr=uint16
  Set_LeftTurnLamp : Outport
  Set_RightTurnLamp : Outport  Port=2
  TurnLightFlashNumberCnt : Outport  Port=3
  wires:
  Constant/1 -> Set_LeftTurnLamp/1
  Constant1/1 -> Set_RightTurnLamp/1
  Constant2/1 -> TurnLightFlashNumberCnt/1

== system DareLib/Dare/Set_TurnLeftRightLampFlash/LeftRightLamp/ON ==
  TurnLightSelect : Inport
  TurnLightFlash_Period : Inport  Port=2
  TurnLightFlash_halfPeriod : Inport  Port=3
  Enable : EnablePort  StatesWhenEnabling=reset
      settings: AttributesFormatString=%<StatesWhenEnabling>
  Set_TurnLampFlash : $bdroot/Dare/Set_TurnLampFlash  TurnLight_Left=1  TurnLight_Right=2  TurnLight_LeftRight=3
  Set_LeftTurnLamp : Outport
  Set_RightTurnLamp : Outport  Port=2
  TurnLightFlashNumberCnt : Outport  Port=3
  wires:
  TurnLightSelect/1 -> Set_TurnLampFlash/1
  TurnLightFlash_Period/1 -> Set_TurnLampFlash/2
  TurnLightFlash_halfPeriod/1 -> Set_TurnLampFlash/3
  Set_TurnLampFlash/1 -> Set_LeftTurnLamp/1
  Set_TurnLampFlash/2 -> Set_RightTurnLamp/1
  Set_TurnLampFlash/3 -> TurnLightFlashNumberCnt/1

== system DareLib/Dare/Set_TurnLeftRightLampFlash/RightLamp/OFF ==
  Enable : EnablePort
  Constant : Constant  Value=0  OutDataTypeStr=uint8
  Constant1 : Constant  Value=0  OutDataTypeStr=uint8
  Constant2 : Constant  Value=0  OutDataTypeStr=uint16
  Set_LeftTurnLamp : Outport
  Set_RightTurnLamp : Outport  Port=2
  TurnLightFlashNumberCnt : Outport  Port=3
  wires:
  Constant/1 -> Set_LeftTurnLamp/1
  Constant1/1 -> Set_RightTurnLamp/1
  Constant2/1 -> TurnLightFlashNumberCnt/1

== system DareLib/Dare/Set_TurnLeftRightLampFlash/RightLamp/ON ==
  TurnLightSelect : Inport
  TurnLightFlash_Period : Inport  Port=2
  TurnLightFlash_halfPeriod : Inport  Port=3
  Enable : EnablePort  StatesWhenEnabling=reset
      settings: AttributesFormatString=%<StatesWhenEnabling>
  Set_TurnLampFlash : $bdroot/Dare/Set_TurnLampFlash  TurnLight_Left=1  TurnLight_Right=2  TurnLight_LeftRight=3
  Set_LeftTurnLamp : Outport
  Set_RightTurnLamp : Outport  Port=2
  TurnLightFlashNumberCnt : Outport  Port=3
  wires:
  TurnLightSelect/1 -> Set_TurnLampFlash/1
  TurnLightFlash_Period/1 -> Set_TurnLampFlash/2
  TurnLightFlash_halfPeriod/1 -> Set_TurnLampFlash/3
  Set_TurnLampFlash/1 -> Set_LeftTurnLamp/1
  Set_TurnLampFlash/2 -> Set_RightTurnLamp/1
  Set_TurnLampFlash/3 -> TurnLightFlashNumberCnt/1

== stateflow chart DareLib/Dare/Set_TurnLampFlash/Set_TurnLampFlash ==
  state [Left,Right]=Set_TurnLamp(OutPutReq,LampSelect) [function]
    (default) -> (junction 61)
    (junction 61) -> (junction 62) [order 1] : [LampSelect == enTurnLight_Left]
    (junction 61) -> (junction 65) [order 2]
    (junction 62) -> (junction 63) : {Left = OutPutReq;}
    (junction 63) -> (junction 64)
    (junction 64) -> (junction 68)
    (junction 65) -> (junction 66) [order 1] : [LampSelect == enTurnLight_Right]
    (junction 65) -> (junction 69) [order 2]
    (junction 66) -> (junction 67) : {Right = OutPutReq;}
    (junction 67) -> (junction 68)
    (junction 68) -> (junction 72)
    (junction 69) -> (junction 70) [order 1] : [LampSelect == enTurnLight_LeftRight]
    (junction 70) -> (junction 71) : {Left = OutPutReq;
        | Right = OutPutReq;}
    (junction 69) -> (junction 73) [order 2] : {Left = 0;
        | Right = 0;}
    (junction 71) -> (junction 72)
    (junction 72) -> (junction 74)
    (junction 74) -> (junction 73)
    (junction 73) -> (junction 75)
  (default) -> (junction 1) : {TurnLightFlashTimeCnt++;}
  (junction 1) -> (junction 3) [order 1] : [TurnLightFlashTimeCnt <= TurnLightFlash_halfPeriod]
  (junction 1) -> (junction 9) [order 2]
  (junction 3) -> (junction 27) : {[Set_LeftTurnLamp,Set_RightTurnLamp] = ...
      |  Set_TurnLamp(ON,TurnLampSelect);}
  (junction 9) -> (junction 11) [order 1] : [TurnLightFlashTimeCnt < TurnLightFlash_Period]
  (junction 9) -> (junction 16) [order 2] : {
      | [Set_LeftTurnLamp,Set_RightTurnLamp] = ...
      |  Set_TurnLamp(OFF,TurnLampSelect);
      | TurnLightFlashTimeCnt  = 0;
      | TurnLightFlashNumberCnt++;}
  (junction 11) -> (junction 13) : {[Set_LeftTurnLamp,Set_RightTurnLamp] = ...
      |  Set_TurnLamp(OFF,TurnLampSelect);}
  (junction 13) -> (junction 16)
  (junction 27) -> (junction 13)
  (junction 16) -> (junction 29)
  data: OutPutReq function_input uint8; LampSelect function_input uint8; Left function_output uint8; Right function_output uint8; TurnLampSelect input; TurnLightFlash_Period input; TurnLightFlash_halfPeriod input; enTurnLight_Left input; enTurnLight_Right input; enTurnLight_LeftRight input; Set_LeftTurnLamp output uint8; Set_RightTurnLamp output uint8; OFF parameter; ON parameter; TurnLightFlashNumberCnt output uint16; TurnLightFlashTimeCnt local uint16

== stateflow chart DareLib/Dare/OutPutMaxTime/Chart ==
  (default) -> (junction 16) : {
      | TargetOutput   = CurrentOutput[0];
      | TargetOutput1 = CurrentOutput[1];
      | TargetOutput2 = CurrentOutput[2];
      | }
  (junction 16) -> (junction 1) [order 1] : [UserModeFlg == 0 && CurrentOutput[0] != UnVaildValue]
  (junction 16) -> (junction 3) [order 2] : {NotUserModeCnt = 0;}
  (junction 1) -> (junction 9)
  (junction 9) -> (junction 2) [order 1] : [NotUserModeCnt < ManufMaxTimPrm]
  (junction 9) -> (junction 18) [order 2] : {TargetOutput = UnVaildValue;}
  (junction 2) -> (junction 14) : {NotUserModeCnt++;}
  (junction 18) -> (junction 3)
  (junction 14) -> (junction 18)
  (junction 3) -> (junction 46)
  (junction 46) -> (junction 48) [order 1] : [UserModeFlg == 0 && CurrentOutput[1] != UnVaildValue]
  (junction 46) -> (junction 50) [order 2] : {NotUserModeCnt1 = 0;}
  (junction 48) -> (junction 43)
  (junction 43) -> (junction 41) [order 1] : [NotUserModeCnt1 < ManufMaxTimPrm]
  (junction 43) -> (junction 35) [order 2] : {TargetOutput1 = UnVaildValue;}
  (junction 41) -> (junction 38) : {NotUserModeCnt1++;}
  (junction 35) -> (junction 50)
  (junction 38) -> (junction 35)
  (junction 50) -> (junction 57)
  (junction 57) -> (junction 56) [order 1] : [UserModeFlg == 0 && CurrentOutput[2] != UnVaildValue]
  (junction 57) -> (junction 67) [order 2] : {NotUserModeCnt2 = 0;}
  (junction 56) -> (junction 70)
  (junction 70) -> (junction 61) [order 1] : [NotUserModeCnt2 < ManufMaxTimPrm]
  (junction 70) -> (junction 60) [order 2] : {TargetOutput2 = UnVaildValue;}
  (junction 61) -> (junction 68) : {NotUserModeCnt2++;}
  (junction 60) -> (junction 67)
  (junction 68) -> (junction 60)
  (junction 67) -> (junction 66)
  data: UserModeFlg input; CurrentOutput input; ManufMaxTimPrm input; UnVaildValue input; TargetOutput output uint8; NotUserModeCnt local uint32; TargetOutput1 output uint8; TargetOutput2 output uint8; NotUserModeCnt1 local uint32; NotUserModeCnt2 local uint32

== stateflow chart DareLib/Dare/SwitchChange/ButtonChange ==
  state NoChange
    en:
    SwSts = enSw_NoChanged;
  state YesChange
    YesChange -> (junction 8) [order 1]
    (default) -> (junction 8)
    (junction 8) -> (junction 10) [order 1] : [PreSw == Vaild_Vaule]
    (junction 8) -> (junction 15) [order 2] : {SwSts = enSw_UnvalidToValid;}
    (junction 10) -> (junction 12) : {SwSts = enSw_ValidToUnvalid;}
    (junction 12) -> (junction 15)
    (junction 15) -> (junction 18) : {PreSw = CurSw;}
  (default) -> NoChange
  NoChange -> YesChange : [PreSw != CurSw && (PreSw == Vaild_Vaule || CurSw == Vaild_Vaule)]
  YesChange -> NoChange [order 1] : [PreSw == CurSw]
  data: CurSw input; enSw_NoChanged input; enSw_UnvalidToValid input; enSw_ValidToUnvalid input; SwSts output uint8; PreSw local uint8; Vaild_Vaule input uint8

== stateflow chart DareLib/Dare/CalCarSpdCondition/Chart ==
  state UpDn
    en:
    VehSpdUpDnFlg = 0;
    UpFlg = 0;
    DnFlg = 0;
    UpCnt = 0;
    DnCnt = 0;
    UpDn -> (junction 135) : {
        | VehSpdUpDnFlg = 0;
        | }
    (default) -> (junction 135)
    (junction 135) -> (junction 132) [order 1] : [VehSpd >= UpVal]
    (junction 135) -> (junction 133) [order 2]
    (junction 132) -> (junction 156) : {UpFlg = 1;}
    (junction 156) -> (junction 133)
    (junction 133) -> (junction 158)
    (junction 158) -> (junction 183) [order 1] : [VehSpd <= DnVal]
    (junction 158) -> (junction 166) [order 2]
    (junction 183) -> (junction 184) : {DnFlg = 1;}
    (junction 184) -> (junction 166)
    (junction 166) -> (junction 162)
    (junction 162) -> (junction 182) [order 1] : [VehSpd < DnVal && UpFlg == 1 && DnFlg == 1]
    (junction 162) -> (junction 136) [order 2]
    (junction 182) -> (junction 163) : {UpCnt = 0;}
    (junction 163) -> (junction 138) [order 1] : [DnCnt < CAL_MaxOnTimer]
    (junction 163) -> (junction 168) [order 2] : {
        | VehSpdUpDnFlg = 1;
        | UpFlg = 0;
        | DnFlg = 0;
        | }
    (junction 138) -> (junction 144) : {DnCnt++;}
    (junction 168) -> (junction 136)
    (junction 144) -> (junction 168)
    (junction 136) -> (junction 139)
    (junction 139) -> (junction 147) [order 1] : [VehSpd > UpVal && UpFlg == 1 && DnFlg == 1]
    (junction 139) -> (junction 167) [order 2]
    (junction 147) -> (junction 154) : {DnCnt = 0;}
    (junction 154) -> (junction 142) [order 1] : [UpCnt < CAL_MaxOnTimer]
    (junction 154) -> (junction 164) [order 2] : {
        | VehSpdUpDnFlg = 2;
        | UpFlg = 0;
        | DnFlg = 0;
        | }
    (junction 142) -> (junction 159) : {UpCnt++;}
    (junction 164) -> (junction 167)
    (junction 159) -> (junction 164)
    (junction 167) -> (junction 169)
  (default) -> UpDn
  data: VehSpd input; DnVal input; UpVal input; CAL_MaxOnTimer input; VehSpdUpDnFlg output uint8; DnCnt local uint32; DnFlg local uint8; UpCnt local uint32; UpFlg local uint8

== stateflow chart DareLib/Dare/Set_SendTimes/Chart ==
  state Clear_OutputData
    en:
    Cnt = 0;
    OutputData = 0;
  state OutPut_Times
    en:
    OutputData = Inputdata;
    Cnt++;
    du:
    Cnt++;
  (default) -> Clear_OutputData
  Clear_OutputData -> OutPut_Times : [hasChanged(Inputdata) && Inputdata != 0]
  OutPut_Times -> Clear_OutputData [order 2] : [Inputdata == 0]
  OutPut_Times -> Clear_OutputData [order 1] : [Cnt >= Times]
  data: Inputdata input; Times input; OutputData output uint8; Cnt local uint16
